simulink model "DeadbeatModel"  (R2018a)
settings: Solver=ode45  StartTime=0.0  StopTime=10*Ts  RelTol=1e-3  SampleTimeConstraint=Specified  EnableMultiTasking=on
values from neighbouring files (symbols this model uses):
  T = 0.01    [FurutaPendulum.m]
undefined symbols (not defined in the file or in its folder): DEN_Gc, DEN_Gp, DEN_GZAS, NUM_Gc, NUM_Gp, NUM_GZAS
settings Model: Creator=James Carroll  LastModifiedBy=Jack
settings DataIOCC: LimitDataPoints=on  SaveFormat=Array  SignalLoggingSaveFormat=ModelDataLogs
settings OptimizationCC: ExpressionDepthLimit=2147483647  InitFltsAndDblsToZero=on  LifeSpan=inf
settings DebuggingCC: UnderspecifiedInitializationDetection=Classic  MergeDetectMultiDrivingBlocksExec=none  FcnCallInpInsideContextMsg=warning  StateNameClashWarn=warning  SFUnexpectedBacktrackingDiag=warning  SFNoUnconditionalDefaultTransitionDiag=warning  SFExecutionAtInitializationDiag=none
settings HardwareCC: ProdBitPerPointer=32  ProdBitPerSizeT=32  ProdBitPerPtrDiffT=32  ProdLargestAtomicFloat=None  ProdIntDivRoundTo=Undefined  ProdEndianess=Unspecified  ProdWordSize=32  ProdHWDeviceType=32-bit Generic
settings ModelReferenceCC: PropagateSignalLabelsOutOfModel=off
settings CodeAppCC: StateflowObjectComments=on
settings GRTTargetCC: TargetLangStandard=C89/C90 (ANSI)  CombineOutputUpdateFcns=off  GRTInterface=on
settings ConfigComp: CovMetricSettings=dw  CovHtmlReporting=on  CovSaveCumulativeToWorkspaceVar=on  CovSaveSingleToWorkspaceVar=on  CovExternalEMLEnable=off

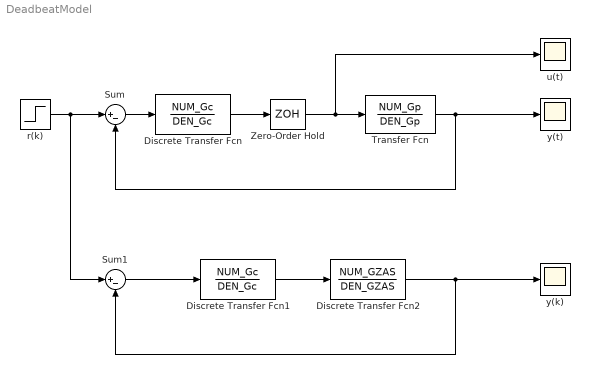
== system DeadbeatModel ==
  Discrete Transfer Fcn : DiscreteTransferFcn  Numerator=NUM_Gc  Denominator=DEN_Gc  SampleTime=T
  Discrete Transfer Fcn1 : DiscreteTransferFcn  Numerator=NUM_Gc  Denominator=DEN_Gc  SampleTime=T
  Discrete Transfer Fcn2 : DiscreteTransferFcn  Numerator=NUM_GZAS  Denominator=DEN_GZAS  SampleTime=T
  Sum : Sum  Inputs=|+-  SampleTime=T
  Sum1 : Sum  Inputs=|+-  SampleTime=T
  Transfer Fcn : TransferFcn  Numerator=NUM_Gp  Denominator=DEN_Gp
  Zero-Order Hold : ZeroOrderHold  SampleTime=T
  r(k) : Step  Time=0  SampleTime=T
  u(t) : Scope
  y(k) : Scope
  y(t) : Scope
  wires:
  Sum/1 -> Discrete Transfer Fcn/1
  r(k)/1 -> Sum/1, Sum1/1
  Transfer Fcn/1 -> Sum/2, y(t)/1
  Discrete Transfer Fcn/1 -> Zero-Order Hold/1
  Zero-Order Hold/1 -> Transfer Fcn/1, u(t)/1
  Sum1/1 -> Discrete Transfer Fcn1/1
  Discrete Transfer Fcn2/1 -> Sum1/2, y(k)/1
  Discrete Transfer Fcn1/1 -> Discrete Transfer Fcn2/1
